simulink subsystem "ApplicationMotorSwapHighPrio"  (R2024b)
settings: Solver=VariableStepAuto  StartTime=0.0  StopTime=10.0  RelTol=1e-3
values from neighbouring files (symbols this model uses):
  Ts = T_pwm    [mcbMotorSwapData.m]
undefined symbols (not defined in the file or in its folder): inverter, NumBits1, NumBits2, Per, pmsm, PosRange1, PosRange2, Slope1, Slope2, Unit
libraries: simulink x17, mcbcontrolslib x4, mcbpmsmparamestlib x3, mcbfoclib x2, mcbpmsmiflib x2, mcbpositiondecoderlib x2, mcbcomputeparameterlib x1, mcbcontrollergainlib x1
(part 2 of 2)

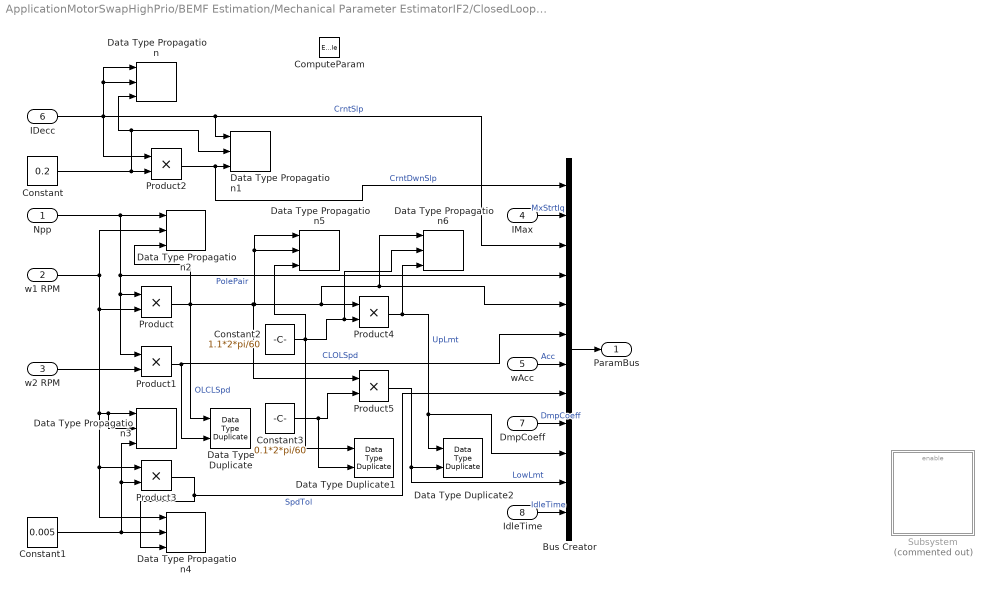
== system ApplicationMotorSwapHighPrio/BEMF Estimation/Mechanical Parameter EstimatorIF2/ClosedLoopFOC/Subsystem1 ==
  Npp : Inport
  w1 RPM : Inport  Port=2
  w2 RPM : Inport  Port=3
  IMax : Inport  Port=4
  wAcc : Inport  Port=5
  IDecc : Inport  Port=6
  DmpCoeff : Inport  Port=7
  IdleTime : Inport  Port=8
  ComputeParam : EnablePort
  Bus Creator : BusCreator  Inputs=12
  Constant : Constant  Value=0.2  OutDataTypeStr=Inherit: Inherit via back propagation  SampleTime=-1
  Constant1 : Constant  Value=0.005  OutDataTypeStr=Inherit: Inherit via back propagation  SampleTime=-1
  Constant2 : Constant  Value=1.1*2*pi/60  OutDataTypeStr=Inherit: Inherit via back propagation  SampleTime=-1
  Constant3 : Constant  Value=0.1*2*pi/60  OutDataTypeStr=Inherit: Inherit via back propagation  SampleTime=-1
  Data Type Duplicate : DataTypeDuplicate
  Data Type Duplicate1 : DataTypeDuplicate
  Data Type Duplicate2 : DataTypeDuplicate
  Data Type Propagation : simulink/Signal Attributes/Data Type Propagation  PropDataType=fixdt(1, 16)  IfRefDouble=double  IfRefSingle=single  IsSigned=IsSigned1 or IsSigned2  NumBitsBase=max([NumBits1 NumBits2])  NumBitsMult=1  NumBitsAdd=0  NumBitsAllowFinal=-1  PropScalingMode=Obtain via best precision  PropScaling=2^-10  ValuesUsedBestPrec=[1 -1]  SlopeBase=min([Slope1 Slope2])  SlopeMult=1  SlopeAdd=0  BiasBase=Bias1  BiasMult=1  BiasAdd=0
  Data Type Propagation{1..2,4,6} (4 alike) : simulink/Signal Attributes/Data Type Propagation  PropDataType=fixdt(1, 16)  IfRefDouble=double  IfRefSingle=single  IsSigned=IsSigned1 or IsSigned2  NumBitsBase=max([NumBits1 NumBits2])  NumBitsMult=1  NumBitsAdd=0  NumBitsAllowFinal=-1  PropScaling=2^-10  ValuesUsedBestPrec=[1 -1]  SlopeBase=PosRange1*PosRange2  SlopeMult=1  SlopeAdd=0  BiasBase=Bias1  BiasMult=1  BiasAdd=0
  Data Type Propagation3 : simulink/Signal Attributes/Data Type Propagation  PropDataType=fixdt(1, 16)  IfRefDouble=double  IfRefSingle=single  IsSigned=IsSigned1 or IsSigned2  NumBitsBase=max([NumBits1 NumBits2])  NumBitsMult=1  NumBitsAdd=0  NumBitsAllowFinal=-1  PropScalingMode=Obtain via best precision  PropScaling=2^-10  ValuesUsedBestPrec=[1 -1]  SlopeBase=min([Slope1 Slope2])  SlopeMult=1  SlopeAdd=0  BiasBase=Bias1  BiasMult=1  BiasAdd=0
  Data Type Propagation5 : simulink/Signal Attributes/Data Type Propagation  PropDataType=fixdt(1, 16)  IfRefDouble=double  IfRefSingle=single  IsSigned=IsSigned1 or IsSigned2  NumBitsBase=max([NumBits1 NumBits2])  NumBitsMult=1  NumBitsAdd=0  NumBitsAllowFinal=-1  PropScalingMode=Obtain via best precision  PropScaling=2^-10  ValuesUsedBestPrec=[1.1*2*pi/60 -1]  SlopeBase=PosRange1*PosRange2  SlopeMult=1  SlopeAdd=0  BiasBase=Bias1  BiasMult=1  BiasAdd=0
  Product{,1..5} (6 alike) : Product  OutDataTypeStr=Inherit: Inherit via back propagation  RndMeth=Simplest
  Subsystem : Subsystem  Commented=on
  ParamBus : Outport
  wires:
  IMax/1 -> Bus Creator/2  "MxStrtIq"
  w1 RPM/1 -> Data Type Propagation2/2, Product/2, Data Type Propagation3/1, Data Type Propagation3/2, Product3/1, Data Type Propagation4/1
  Constant/1 -> Product2/2, Data Type Propagation1/2, Data Type Propagation/3
  IDecc/1 -> Data Type Propagation1/1, Bus Creator/3, Data Type Propagation/1, Data Type Propagation/2, Product2/1  "CrntSlp"
  Product/1 -> Product5/1, Data Type Propagation5/2, Data Type Propagation5/1, Product4/1, Data Type Propagation6/1, Bus Creator/5, Data Type Propagation2/3, Data Type Duplicate/1  "OLCLSpd"
  Constant3/1 -> Product5/2, Data Type Duplicate1/2
  Product2/1 -> Bus Creator/1, Data Type Propagation1/3  "CrntDwnSlp"
  IdleTime/1 -> Bus Creator/12  "IdleTime"
  Constant2/1 -> Product4/2, Data Type Propagation6/2, Data Type Propagation5/3, Data Type Duplicate1/1
  Npp/1 -> Data Type Propagation2/1, Bus Creator/4, Product1/1, Product/1  "PolePair"
  Product1/1 -> Data Type Duplicate/2, Bus Creator/6  "CLOLSpd"
  w2 RPM/1 -> Product1/2
  Bus Creator/1 -> ParamBus/1
  Product5/1 -> Data Type Duplicate2/2, Bus Creator/11  "LowLmt"
  wAcc/1 -> Bus Creator/7  "Acc"
  DmpCoeff/1 -> Bus Creator/9  "DmpCoeff"
  Product3/1 -> Bus Creator/8, Data Type Propagation4/3  "SpdTol"
  Product4/1 -> Data Type Propagation6/3, Bus Creator/10, Data Type Duplicate2/1  "UpLmt"
  Constant1/1 -> Data Type Propagation4/2, Data Type Propagation3/3, Product3/2

== system ApplicationMotorSwapHighPrio/BEMF Estimation/Mechanical Parameter EstimatorIF2/ClosedLoopFOC/Subsystem2 ==
  Debug : Inport
  Ibase : Inport  Port=2
  Vdc : Inport  Port=3
  Gain4 : Gain  Gain=1/sqrt(3)  RndMeth=Simplest  OutDataTypeStr=Inherit: Same as input
  Product : Product
  Product1 : Product
  Selector1 : Selector  InputPortWidth=8  IndexOptions=Index vector (dialog)  Indices=[1 2]  OutputSizes=1
  Selector2 : Selector  InputPortWidth=8  IndexOptions=Index vector (dialog)  Indices=[3 4]  OutputSizes=1
  Selector3 : Selector  InputPortWidth=8  IndexOptions=Index vector (dialog)  Indices=[5 6 7 8]  OutputSizes=1
  Selector4 : Selector  InputPortWidth=2  IndexOptions=Index vector (dialog)  Indices=[2]  OutputSizes=1
  Selector5 : Selector  InputPortWidth=2  IndexOptions=Index vector (dialog)  Indices=[2]  OutputSizes=1
  Idq : Outport
  Vdq : Outport  Port=2
  VIAB : Outport  Port=3
  Iq : Outport  Port=4
  Vq : Outport  Port=5
  wires:
  Selector1/1 -> Idq/1, Selector4/1
  Selector3/1 -> VIAB/1
  Selector5/1 -> Product1/1
  Gain4/1 -> Product1/2
  Selector4/1 -> Product/1
  Vdc/1 -> Gain4/1
  Debug/1 -> Selector1/1, Selector3/1, Selector2/1
  Selector2/1 -> Vdq/1, Selector5/1
  Product/1 -> Iq/1
  Ibase/1 -> Product/2
  Product1/1 -> Vq/1

== system ApplicationMotorSwapHighPrio/FluxObserver/Speed Calculation from Back EMF/Speed Measurement/Enabled Subsystem ==
  In1 : Inport
  Enable : EnablePort
  Add : Sum  Inputs=+-
  Reciprocal : Product  Inputs=/
  Unit Delay : UnitDelay  SampleTime=-1  HasFrameUpgradeWarning=on
  Out1 : Outport
  wires:
  In1/1 -> Add/1, Unit Delay/1
  Unit Delay/1 -> Add/2
  Add/1 -> Reciprocal/1
  Reciprocal/1 -> Out1/1

== system ApplicationMotorSwapHighPrio/FluxObserver/Speed Calculation from Back EMF/Speed Measurement/Up Counter ==
  Enable : EnablePort  StatesWhenEnabling=reset
  Add1 : Sum  SaturateOnIntegerOverflow=on
  Constant : Constant  OutDataTypeStr=uint32
  Delay : Delay  DelayLength=1
  Count : Outport  OutputWhenDisabled=reset  InitialOutput=0
  wires:
  Delay/1 -> Add1/2
  Add1/1 -> Count/1, Delay/1
  Constant/1 -> Add1/1

== system ApplicationMotorSwapHighPrio/BEMF Estimation/Mechanical Parameter EstimatorIF2/ClosedLoopFOC/Subsystem1/Subsystem ==
  Enable : EnablePort
  Compute Parameter : mcbcomputeparameterlib/Compute Parameter  Commented=on  PathOfCompatibleBlock=Microcontroller/ApplicationFastTask/BEMF Estimation/Mechanical Parameter EstimatorIF2/ClosedLoopFOC/I-F Controller

== stateflow chart ApplicationMotorSwapHighPrio/BEMF Estimation/Mechanical Parameter EstimatorIF2/Test Control Stateflow/Stateflow ==
  state Init
    entry:
    ClosedLoopEn = false;
    StatusOut = uint16(0);
    TimelimitTicks = (KeTime + 100)/Ts;
    VabcEn = false;
    CalcParams = false;
    PIGainEn = false;
  state Run
    state Initrun
      entry:
      StatusOut = uint16(1);
    state ComputeParam
      during:
      PIGainEn = true;
    state ClosedLoop
      during:
      PIGainEn = false;
      ClosedLoopEn = true;
      VabcEn = true;
      CalcParams = true;
    state Error
      during:
      StatusOut = uint16(8300);
      VabcEn = false;
      CalcParams = false;
    state InvDisable
      during:
      ClosedLoopEn = false;
      VabcEn = false;
    state Complete
      during:
      StatusOut = uint16(2);
      CalcParams = false;
    (default) -> Initrun
    Initrun -> ComputeParam : [InvEn == true]
    ComputeParam -> (junction 12) [order 1] : after(0.25/Ts, tick)
    ComputeParam -> Error [order 2] : after(TimelimitTicks,tick)
    (junction 12) -> ClosedLoop
    ClosedLoop -> (junction 19) [order 2] : after(TimelimitTicks,tick)
    (junction 19) -> Error
    ClosedLoop -> InvDisable [order 1] : [InvEn == false]
    InvDisable -> Complete : [StatusIn >0]
  (default) -> Init
  Run -> Init : [EnIn == true && EnInPrev == false]
  Init -> Run : [EnIn == true]
  data: VabcEn output; EnIn input; EnInPrev input; StartFOC input; InvEn input; StatusIn input uint16; KeTime input; Ts input; ClosedLoopEn output; CalcParams output; PIGainEn output; StatusOut output; TimelimitTicks local

== matlab function ApplicationMotorSwapHighPrio/BEMF Estimation/Mechanical Parameter EstimatorIF2/Calculate Parameters/MATLAB Function ==
  data: Rs input single; Ke output single; J output single; Ld input single; Id input single; Iq input single; Vd input single; Vq input single; KeTime input single; KeTrigSpeed input single; Ts input single; B output single; Speed input single; PolePairs input single; SpeedLowerLimIntertia input single; inverterEn output single; Status output uint16; CoastDownTime output single
function [Ke, J, B, inverterEn, Status, CoastDownTime]  = fcn(Rs, Ld, Id, Iq, Vd, Vq, KeTime, KeTrigSpeed, Ts, Speed, PolePairs, SpeedLowerLimIntertia)
coder.allowpcode('plain'); 

%#codegen
[Ke, J, B, inverterEn, Status, CoastDownTime] = mcb.internal.estimatePMSMMechanicalParameters(Rs, Ld, Id, Iq, Vd, Vq, KeTime, KeTrigSpeed, Ts, Speed, PolePairs, SpeedLowerLimIntertia);
